simulink model "OMP_with_base"  (R2023b)
settings: Solver=VariableStepAuto  StartTime=0.0  StopTime=100  RelTol=1e-3
libraries: roblocks x2
settings Model: Creator=kangwang  LastModifiedBy=kangwang

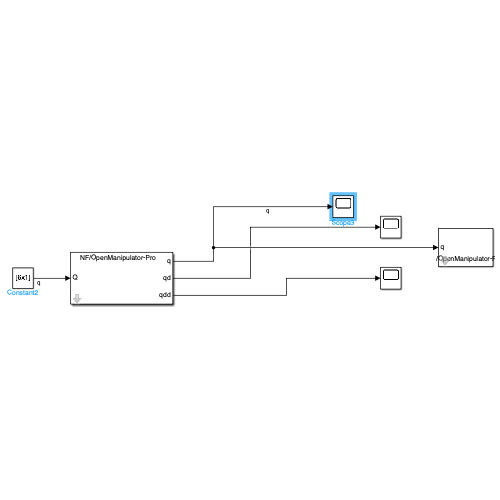
[thumbnail: Simulink's stored preview of the top-level diagram]
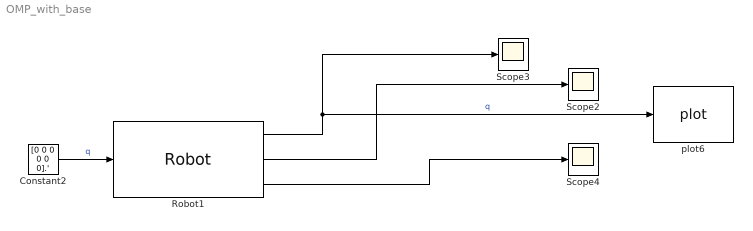
== system OMP_with_base ==
  Constant2 : Constant  Value=[0 0 0 0 0 0].'
  Robot1 : roblocks/Arm/Robot  robot=openmanipulator_pro.nofriction  q0=[0 0 0 0 0 0]
      link override Integrator1: InitialCondition=[0 0 0 0 0 0]
  Scope2 : Scope
  Scope3 : Scope
  Scope4 : Scope
  plot6 : roblocks/Arm/plot  robot=openmanipulator_pro.nofriction  fps=10  holdplot=on
  wires:
  Robot1/3 -> Scope4/1
  Robot1/2 -> Scope2/1
  Constant2/1 -> Robot1/1  "q"
  Robot1/1 -> Scope3/1, plot6/1  "q"
